simulink model "pacejka_lateral_model"  (R2023a)
settings: Solver=FixedStepAuto  StartTime=0.0  StopTime=10.0  FixedStep=0.01  RelTol=1e-3
values from neighbouring files (symbols this model uses):
  a1F = -1e-05    [formulacar_params.mat]
  a1R = -1e-05    [formulacar_params.mat]
  a2F = 1.25    [formulacar_params.mat]
  a2R = 1.25    [formulacar_params.mat]
  BF = 0.2719    [formulacar_params.mat]
  BR = 0.3609    [formulacar_params.mat]
  CF = 1.8391    [formulacar_params.mat]
  CR = 1.7631    [formulacar_params.mat]
  EF = -2.5276    [formulacar_params.mat]
  ER = -1.989    [formulacar_params.mat]
  FzF = 4463.32301587    [formulacar_params.mat]
  FzR = 4725.87142857    [formulacar_params.mat]
settings Model: Creator=Cassio.Freitas  LastModifiedBy=Cassio de Freitas
settings SolverCC: AlgebraicLoopSolver=TrustRegion
settings DataIOCC: ReturnWorkspaceOutputs=off
settings DebuggingCC: UnconnectedInputMsg=warning  UnconnectedOutputMsg=warning  UnconnectedLineMsg=warning  ArithmeticOperatorsInVariantConditions=warning
settings ModelReferenceCC: EnableRefExpFcnMdlSchedulingChecks=on
settings SFSimCC: CustomCodeUndefinedFunction=UseInterfaceOnly

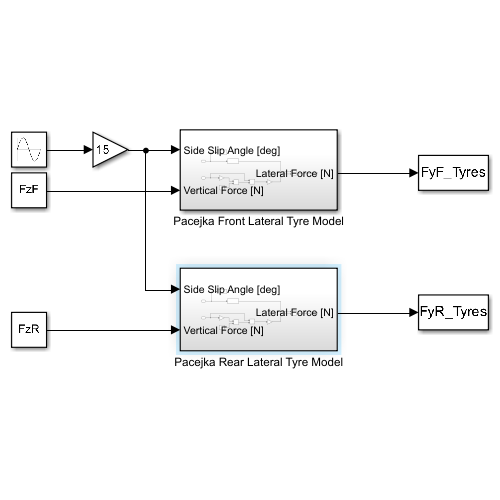
[thumbnail: Simulink's stored preview of the top-level diagram]
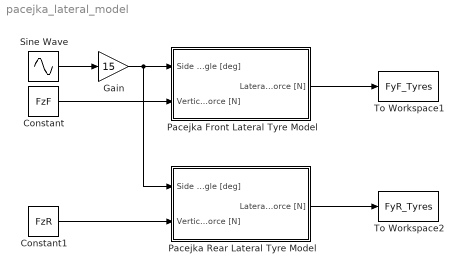
== system pacejka_lateral_model ==
  Constant : Constant  Value=FzF
  Constant1 : Constant  Value=FzR
  Gain : Gain  Gain=15
  Pacejka Front Lateral Tyre Model : Subsystem
  Pacejka Rear Lateral Tyre Model : Subsystem
  Sine Wave : Sin  SampleTime=0
  To Workspace1 : ToWorkspace  VariableName=FyF_Tyres  SaveFormat=Timeseries  SampleTime=-1
  To Workspace2 : ToWorkspace  VariableName=FyR_Tyres  SaveFormat=Timeseries  SampleTime=-1
  wires:
  Constant/1 -> Pacejka Front Lateral Tyre Model/2(Vertical Force [N])
  Sine Wave/1 -> Gain/1
  Gain/1 -> Pacejka Rear Lateral Tyre Model/1(Side Slip Angle [deg]), Pacejka Front Lateral Tyre Model/1(Side Slip Angle [deg])
  Pacejka Front Lateral Tyre Model/1(Lateral Force [N]) -> To Workspace1/1
  Pacejka Rear Lateral Tyre Model/1(Lateral Force [N]) -> To Workspace2/1
  Constant1/1 -> Pacejka Rear Lateral Tyre Model/2(Vertical Force [N])

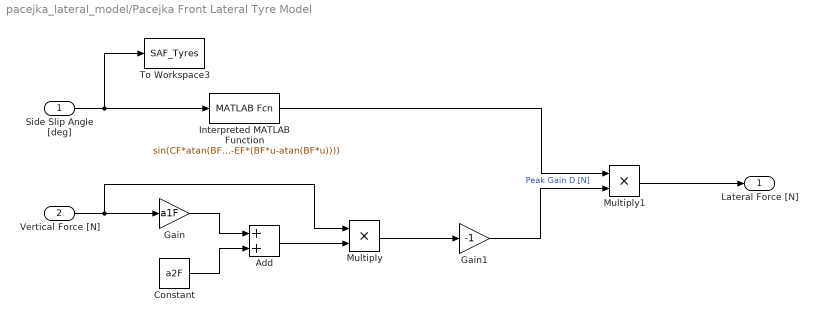
== system pacejka_lateral_model/Pacejka Front Lateral Tyre Model ==
  Side Slip Angle [deg] : Inport
  Vertical Force [N] : Inport  Port=2
  Add : Sum
  Constant : Constant  Value=a2F
  Gain : Gain  Gain=a1F
  Gain1 : Gain  Gain=-1
  Interpreted MATLAB Function : MATLABFcn  MATLABFcn=sin(CF*atan(BF*u-EF*(BF*u-atan(BF*u))))
  Multiply : Product
  Multiply1 : Product
  To Workspace3 : ToWorkspace  VariableName=SAF_Tyres  SaveFormat=Timeseries  SampleTime=-1
  Lateral Force [N] : Outport  VectorParamsAs1DForOutWhenUnconnected=off
  wires:
  Vertical Force [N]/1 -> Gain/1, Multiply/1
  Constant/1 -> Add/2
  Gain/1 -> Add/1
  Add/1 -> Multiply/2
  Multiply/1 -> Gain1/1
  Gain1/1 -> Multiply1/2  "Peak Gain D [N]"
  Side Slip Angle [deg]/1 -> To Workspace3/1, Interpreted MATLAB Function/1
  Interpreted MATLAB Function/1 -> Multiply1/1
  Multiply1/1 -> Lateral Force [N]/1

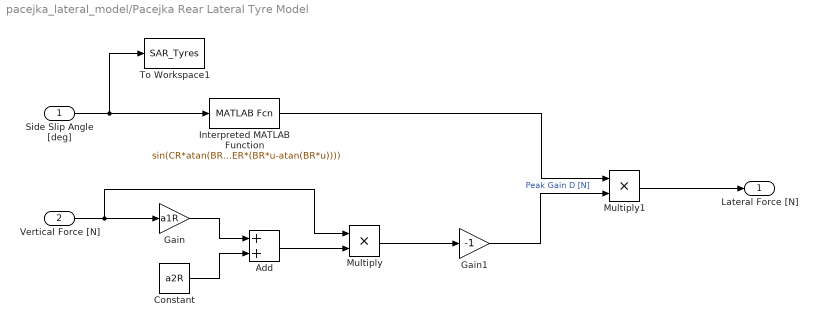
== system pacejka_lateral_model/Pacejka Rear Lateral Tyre Model ==
  Side Slip Angle [deg] : Inport
  Vertical Force [N] : Inport  Port=2
  Add : Sum
  Constant : Constant  Value=a2R
  Gain : Gain  Gain=a1R
  Gain1 : Gain  Gain=-1
  Interpreted MATLAB Function : MATLABFcn  MATLABFcn=sin(CR*atan(BR*u-ER*(BR*u-atan(BR*u))))
  Multiply : Product
  Multiply1 : Product
  To Workspace1 : ToWorkspace  VariableName=SAR_Tyres  SaveFormat=Timeseries  SampleTime=-1
  Lateral Force [N] : Outport  VectorParamsAs1DForOutWhenUnconnected=off
  wires:
  Interpreted MATLAB Function/1 -> Multiply1/1
  Side Slip Angle [deg]/1 -> To Workspace1/1, Interpreted MATLAB Function/1
  Gain1/1 -> Multiply1/2  "Peak Gain D [N]"
  Multiply/1 -> Gain1/1
  Add/1 -> Multiply/2
  Gain/1 -> Add/1
  Constant/1 -> Add/2
  Vertical Force [N]/1 -> Multiply/1, Gain/1
  Multiply1/1 -> Lateral Force [N]/1
